simulink library "library_IMUPackaging"  (R2024a)
settings: Solver=VariableStepAuto  StartTime=0.0  StopTime=10.0  RelTol=1e-3
libraries: library_IMUPackagingSFunc x1
settings Model: Creator=tommy  LastModifiedBy=tommy

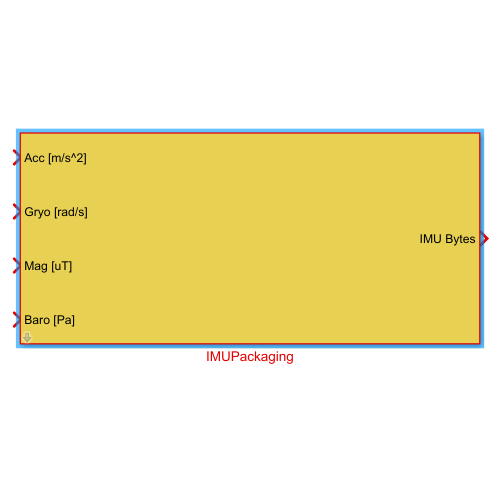
[thumbnail: Simulink's stored preview of the top-level diagram]
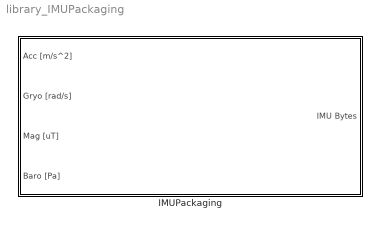
== system library_IMUPackaging ==
  IMUPackaging : Subsystem
      mask help: Default Mask

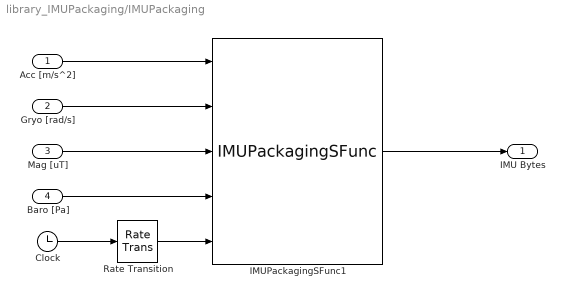
== system library_IMUPackaging/IMUPackaging ==
  Acc [m/s^2] : Inport
  Gryo [rad/s] : Inport  Port=2
  Mag [uT] : Inport  Port=3
  Baro [Pa] : Inport  Port=4
  Clock : Clock
  IMUPackagingSFunc1 : library_IMUPackagingSFunc/IMUPackagingSFunc
  Rate Transition : RateTransition  OutPortSampleTimeOpt=Inherit
  IMU Bytes : Outport
  wires:
  IMUPackagingSFunc1/1 -> IMU Bytes/1
  Acc [m/s^2]/1 -> IMUPackagingSFunc1/1
  Gryo [rad/s]/1 -> IMUPackagingSFunc1/2
  Mag [uT]/1 -> IMUPackagingSFunc1/3
  Baro [Pa]/1 -> IMUPackagingSFunc1/4
  Clock/1 -> Rate Transition/1
  Rate Transition/1 -> IMUPackagingSFunc1/5
